simulink library "control_command_generation_lib"  (R2018b)
settings: Solver=VariableStepAuto  StartTime=0.0  StopTime=10.0  RelTol=1e-3
undefined symbols (not defined in the file): fswParams
libraries: command_converter_lib x1, controlSelection_lib x1, quat_err_lib x1, rwa_allocation_lib x1
settings Model: Creator=colem  LastModifiedBy=Taylor

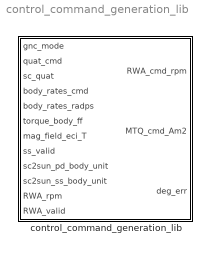
== system control_command_generation_lib ==
  control_command_generation_lib : Subsystem

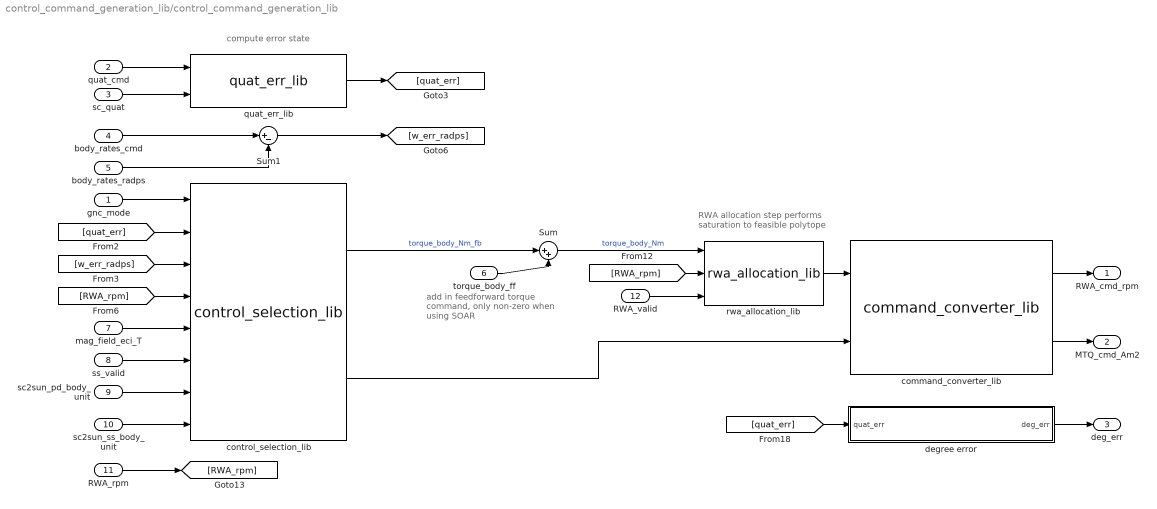
== system control_command_generation_lib/control_command_generation_lib ==
  note: compute error state
  note: RWA allocation step performs
      | saturation to feasible polytope
  note: add in feedforward torque
      | command, only non-zero
      | when using SOAR
  gnc_mode : Inport
  quat_cmd : Inport  Port=2
  sc_quat : Inport  Port=3
  body_rates_cmd : Inport  Port=4
  body_rates_radps : Inport  Port=5
  torque_body_ff : Inport  Port=6
  mag_field_eci_T : Inport  Port=7
  ss_valid : Inport  Port=8
  sc2sun_pd_body_unit : Inport  Port=9
  sc2sun_ss_body_unit : Inport  Port=10
  RWA_rpm : Inport  Port=11
  RWA_valid : Inport  Port=12
  Sum : Sum  Inputs=|++
  Sum1 : Sum  Inputs=|+-
  command_converter_lib : command_converter_lib/command_converter_lib  SystemSampleTime=-1
  control_selection_lib : controlSelection_lib/control_selection_lib  SystemSampleTime=-1
  degree error : Subsystem
  quat_err_lib : quat_err_lib/quat_err_lib  SystemSampleTime=-1
  rwa_allocation_lib : rwa_allocation_lib/rwa_allocation_lib  SystemSampleTime=-1
  RWA_cmd_rpm : Outport
  MTQ_cmd_Am2 : Outport  Port=2
  deg_err : Outport  Port=3
  wires:
  Sum/1 -> rwa_allocation_lib/1  "torque_body_Nm"
  control_selection_lib/2 -> command_converter_lib/2
  mag_field_eci_T/1 -> control_selection_lib/5
  RWA_rpm/1 -> [RWA_rpm]
  quat_cmd/1 -> quat_err_lib/1
  sc_quat/1 -> quat_err_lib/2
  quat_err_lib/1 -> [quat_err]
  [RWA_rpm] -> rwa_allocation_lib/2
  RWA_valid/1 -> rwa_allocation_lib/3
  rwa_allocation_lib/1 -> command_converter_lib/1
  command_converter_lib/1 -> RWA_cmd_rpm/1
  command_converter_lib/2 -> MTQ_cmd_Am2/1
  torque_body_ff/1 -> Sum/2
  gnc_mode/1 -> control_selection_lib/1
  control_selection_lib/1 -> Sum/1  "torque_body_Nm_fb"
  degree error/1(deg_err) -> deg_err/1
  [quat_err] -> degree error/1(quat_err)
  body_rates_radps/1 -> Sum1/2
  body_rates_cmd/1 -> Sum1/1
  Sum1/1 -> [w_err_radps]
  [quat_err] -> control_selection_lib/2
  [w_err_radps] -> control_selection_lib/3
  [RWA_rpm] -> control_selection_lib/4
  sc2sun_ss_body_unit/1 -> control_selection_lib/8
  sc2sun_pd_body_unit/1 -> control_selection_lib/7
  ss_valid/1 -> control_selection_lib/6

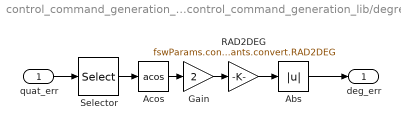
== system control_command_generation_lib/control_command_generation_lib/degree error ==
  quat_err : Inport
  Abs : Abs
  Acos : Trigonometry  Operator=acos
  Gain : Gain  Gain=2
  RAD2DEG : Gain  Gain=fswParams.constants.convert.RAD2DEG
  Selector : Selector  InputPortWidth=4  IndexOptions=Index vector (dialog)  Indices=[1]  OutputSizes=1
  deg_err : Outport
  wires:
  RAD2DEG/1 -> Abs/1
  Gain/1 -> RAD2DEG/1
  Acos/1 -> Gain/1
  Selector/1 -> Acos/1
  Abs/1 -> deg_err/1
  quat_err/1 -> Selector/1
